simulink model "Concatenate_TestGen9"  (R2017b)
settings: Solver=FixedStepDiscrete  StartTime=0.0  StopTime=10.0  RelTol=1e-3
settings Model: Creator=ktrinh  LastModifiedBy=ktrinh
settings DebuggingCC: ParameterOverflowMsg=none

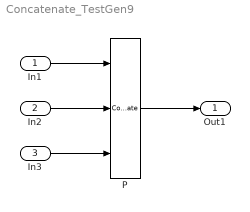
== system Concatenate_TestGen9 ==
  In1 : Inport  OutDataTypeStr=single  PortDimensions=[2 4 5]
  In2 : Inport  Port=2  OutDataTypeStr=single  PortDimensions=[2 4 5]
  In3 : Inport  Port=3  OutDataTypeStr=single  PortDimensions=[2 4 5]
  P : Concatenate  NumInputs=3  Mode=Multidimensional array  ConcatenateDimension=2
  Out1 : Outport
  wires:
  In1/1 -> P/1
  In2/1 -> P/2
  In3/1 -> P/3
  P/1 -> Out1/1
